simulink model "mayhemit"  (R2023b)
settings: Solver=FixedStepAuto  StartTime=0.0  StopTime=10.0  RelTol=1e-3
settings Model: Creator=ubuntu  LastModifiedBy=ubuntu
settings DataIOCC: SaveFormat=Array  SaveOutput=off  SignalLogging=off  DSMLogging=off  StreamToWks=off  SaveTime=off  ReturnWorkspaceOutputs=off  DatasetSignalFormat=timetable
settings OptimizationCC: DefaultParameterBehavior=Inlined  EnhancedBackFolding=on  PassReuseOutputArgsThreshold=0  OptimizeBlockOrder=speed  DifferentSizesBufferReuse=on  OptimizationCustomize=off
settings DebuggingCC: ParameterTunabilityLossMsg=error
settings HardwareCC: ProdBitPerLong=64  ProdHWDeviceType=AMD->x86-64 (Linux 64)  TargetBitPerLong=64  TargetBitPerPointer=64  TargetBitPerSizeT=64  TargetBitPerPtrDiffT=64  TargetLongLongMode=on  TargetIntDivRoundTo=Zero  TargetEndianess=LittleEndian  TargetWordSize=64  TargetHWDeviceType=MATLAB Host  ProdEqTarget=off
settings SFSimCC: MATLABDynamicMemAlloc=off
settings RTWCC: GenCodeOnly=on
settings CodeAppCC: ForceParamTrailComments=on  OperatorAnnotations=on

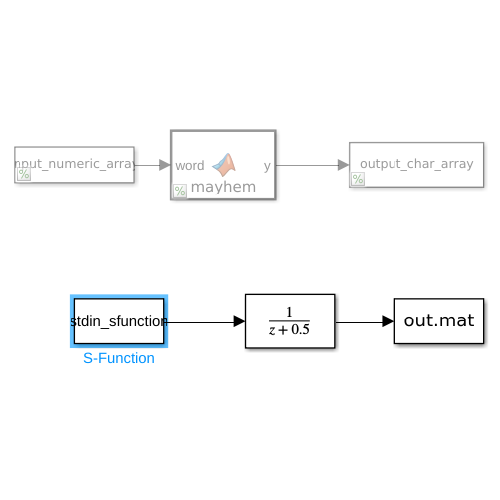
[thumbnail: Simulink's stored preview of the top-level diagram]
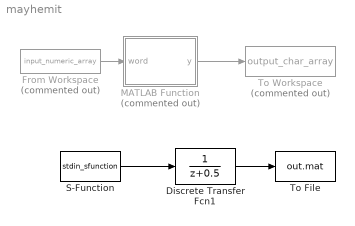
== system mayhemit ==
  Discrete Transfer Fcn1 : DiscreteTransferFcn
  From Workspace : FromWorkspace  Commented=on  VariableName=input_numeric_array
  MATLAB Function : MATLAB Function  Commented=on  TreatAsAtomicUnit=on
  S-Function : S-Function  FunctionName=stdin_sfunction  SFunctionDeploymentMode=off  EnableBusSupport=off
  To File : ToFile  Filename=out.mat
  To Workspace : ToWorkspace  Commented=on  VariableName=output_char_array  SaveFormat=Timeseries  SampleTime=-1
  wires:
  MATLAB Function/1(y) -> To Workspace/1
  From Workspace/1 -> MATLAB Function/1(word)
  Discrete Transfer Fcn1/1 -> To File/1
  S-Function/1 -> Discrete Transfer Fcn1/1

== matlab function mayhemit/MATLAB Function ==
  data: word input; y output
function y = mayhem(word)
    word = char(word);
    
    % Check if the input is a char array
    assert(ischar(word), 'Input must be a char array or string.');
 
    if length(word) >= 1 && word(1) == 'b'
        if length(word) >= 2 && word(2) == 'u'
            if length(word) >= 3 && word(3) == 'g'
                fprintf('Bug here!\n');
                len = 1e7;
                for i = 1:len
                    m = mod(length(word), i) + 1;
                    word(i) = word(m);
                end
            end
        end
    end
    fprintf('%s\n', word);
    y = double(word);
end
